simulink model "PID_discrete"  (R2021b)
settings: Solver=VariableStepAuto  StartTime=0.0  StopTime=50  RelTol=1e-3
values from neighbouring files (symbols this model uses):
  T = 0.001    [c_controller_designer.m]    (also in control_design_mat.m = 0.0005)
undefined symbols (not defined in the file or in its folder): a_ac, a_dd, a_pid, b_ac, b_dd, b_pid, param
libraries: simulink x1
settings Model: Creator=Natalie  LastModifiedBy=Trevor

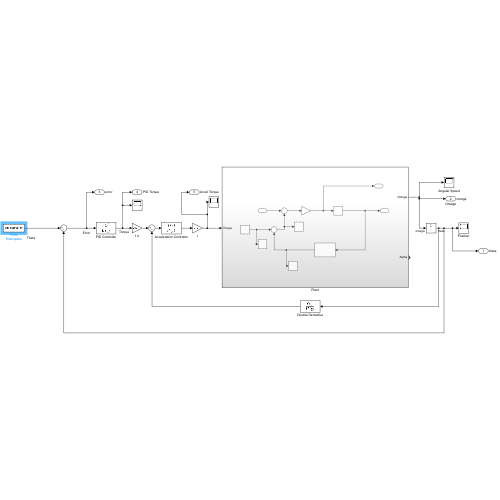
[thumbnail: Simulink's stored preview of the top-level diagram]
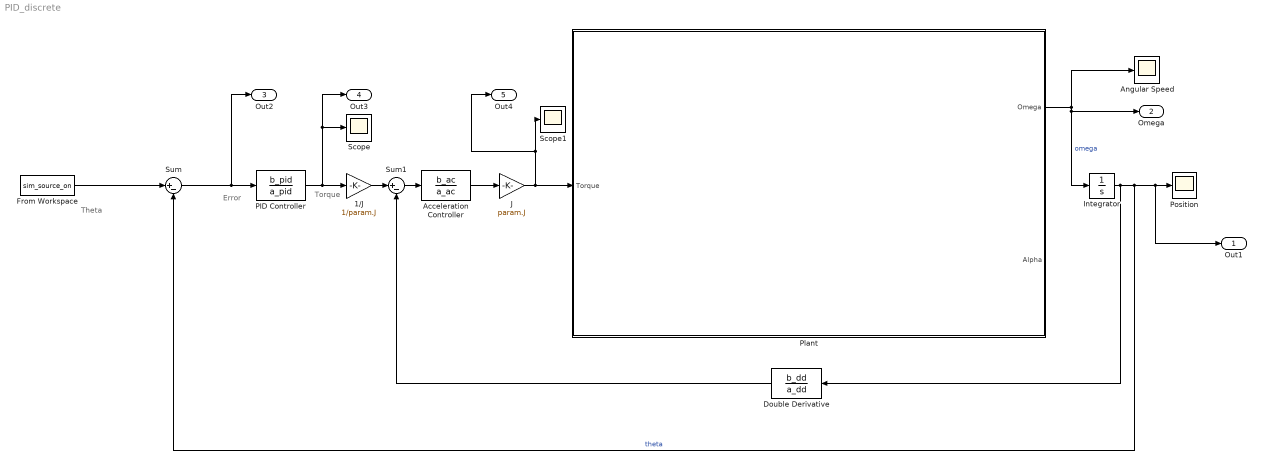
== system PID_discrete ==
  note: Torque
  note: Error
  note: Theta
  1/J : Gain  Gain=1/param.J
  Acceleration Controller : DiscreteTransferFcn  Numerator=b_ac  Denominator=a_ac  SampleTime=T
  Angular Speed : Scope
  Double Derivative : DiscreteTransferFcn  Numerator=b_dd  Denominator=a_dd  SampleTime=T
  From Workspace : FromWorkspace  VariableName=sim_source_on
  Integrator : Integrator
  J : Gain  Gain=param.J
  PID Controller : DiscreteTransferFcn  Numerator=b_pid  Denominator=a_pid  SampleTime=T
  Plant : Subsystem
  Position : Scope
  Scope : Scope
  Scope1 : Scope
  Sum : Sum  Inputs=|+-
  Sum1 : Sum  Inputs=|+-
  Out1 : Outport  SignalName=theta
  Omega : Outport  Port=2  SignalName=omega
  Out2 : Outport  Port=3  SignalName=error
  Out3 : Outport  Port=4  SignalName=PID Torque
  Out4 : Outport  Port=5  SignalName=Accel Torque
  wires:
  Plant/1(Omega) -> Integrator/1, Omega/1, Angular Speed/1  "omega"
  Integrator/1 -> Double Derivative/1, Out1/1, Position/1, Sum/2  "theta"
  From Workspace/1 -> Sum/1
  Sum/1 -> PID Controller/1, Out2/1
  PID Controller/1 -> 1/J/1, Scope/1, Out3/1
  1/J/1 -> Sum1/1
  J/1 -> Out4/1, Scope1/1, Plant/1(Torque)
  Sum1/1 -> Acceleration Controller/1
  Acceleration Controller/1 -> J/1
  Double Derivative/1 -> Sum1/2

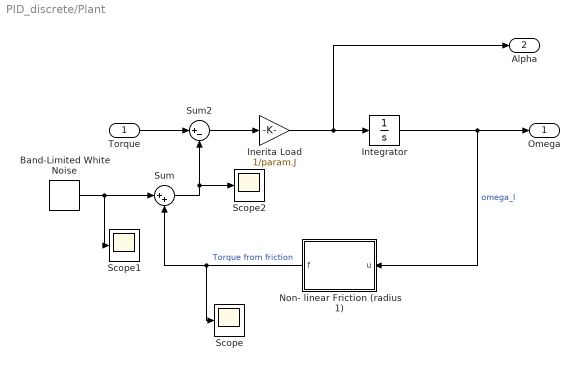
== system PID_discrete/Plant ==
  Torque : Inport
  Band-Limited White Noise : simulink/Sources/Band-Limited White Noise  Cov=[0]  Ts=0.0042  seed=[23341]
  Inerita Load : Gain  Gain=1/param.J
  Integrator : Integrator
  Non- linear Friction (radius 1) : MATLAB Function  TreatAsAtomicUnit=on
  Scope : Scope
  Scope1 : Scope
  Scope2 : Scope
  Sum : Sum  Inputs=|++
  Sum2 : Sum  Inputs=|+-
  Omega : Outport
  Alpha : Outport  Port=2
  wires:
  Integrator/1 -> Omega/1, Non- linear Friction (radius 1)/1(u)  "omega_l"
  Non- linear Friction (radius 1)/1(f) -> Sum/2, Scope/1  "Torque from friction"
  Torque/1 -> Sum2/1
  Sum2/1 -> Inerita Load/1
  Inerita Load/1 -> Alpha/1, Integrator/1
  Band-Limited White Noise/1 -> Scope1/1, Sum/1
  Sum/1 -> Scope2/1, Sum2/2

== matlab function PID_discrete/Plant/Non- linear Friction (radius 1) ==
  data: u input; f output; param parameter

function f = friction_m(u, param)

%FRICTION_M Nonlinear friction model with Stribeck, Coulomb and viscous

% dissipation effects.

% Output equation.

f = param.g1*(tanh(param.g2*u)-tanh(param.g3*u)) ... % Stribeck effect.
+ param.g4*tanh(param.g5*u) ... % Coulomb effect.
+ param.g6*u; % Viscous dissipation term.

end
